simulink model "inverse_kinematics_simulation_with_y_pose"  (R2014a)
settings: Solver=ode45  StartTime=0.0  StopTime=inf  RelTol=1e-3
values from neighbouring files (symbols this model uses):
  h1 = y(:,1)    [initial_conditions.m]    (also in inverse_kinematics.m)
  h2 = z(:,2)    [initial_conditions.m]    (also in inverse_kinematics.m)
  h3 = x(:,3)    [initial_conditions.m]    (also in inverse_kinematics.m)
  h4 = z(:,4)    [initial_conditions.m]    (also in inverse_kinematics.m)
  h5 = x(:,5)    [initial_conditions.m]    (also in inverse_kinematics.m)
  h6 = x(:,6)    [initial_conditions.m]    (also in inverse_kinematics.m)
  h7 = y(:,7)    [initial_conditions.m]    (also in inverse_kinematics.m)
  sampling_time = 0.01    [initial_conditions.m]
libraries: vrlib x1
settings Model: Creator=İSMAİL  LastModifiedBy=İSMAİL

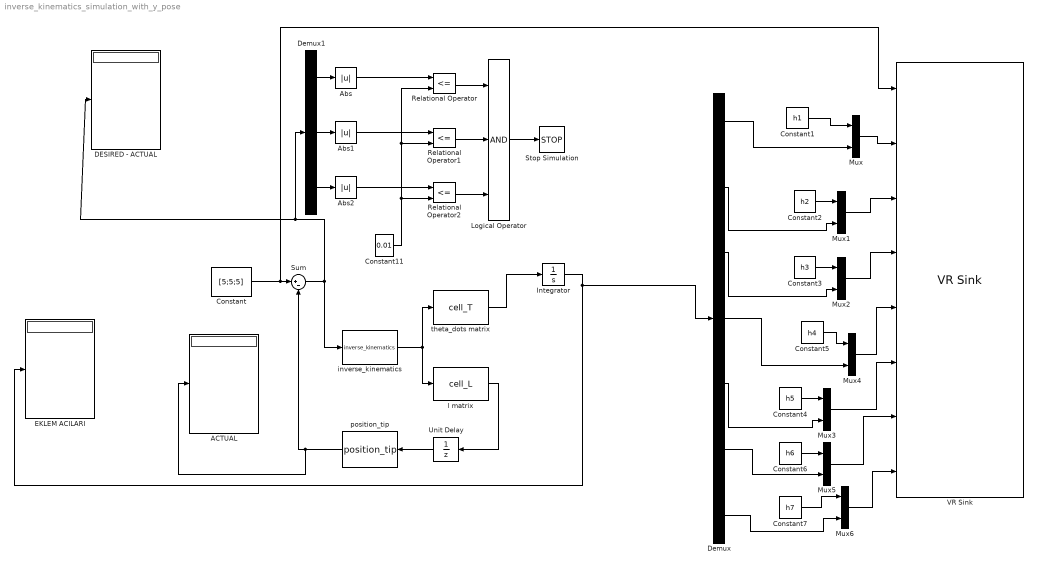
== system inverse_kinematics_simulation_with_y_pose ==
  ACTUAL : Display
  Abs : Abs
  Abs1 : Abs
  Abs2 : Abs
  Constant : Constant  Value=[5;5;5]  VectorParams1D=off
  Constant1 : Constant  Value=h1  VectorParams1D=off
  Constant11 : Constant  Value=0.01  VectorParams1D=off
  Constant2 : Constant  Value=h2  VectorParams1D=off
  Constant3 : Constant  Value=h3  VectorParams1D=off
  Constant4 : Constant  Value=h5  VectorParams1D=off
  Constant5 : Constant  Value=h4  VectorParams1D=off
  Constant6 : Constant  Value=h6  VectorParams1D=off
  Constant7 : Constant  Value=h7  VectorParams1D=off
  DESIRED - ACTUAL : Display
  Demux : Demux  Outputs=7
  Demux1 : Demux  Outputs=3
  EKLEM ACILARI : Display
  Integrator : Integrator
  Logical Operator : Logic  Inputs=3  AllPortsSameDT=off  OutDataTypeStr=boolean
  Mux{,1..6} (7 alike) : Mux  Inputs=2
  Relational Operator : RelationalOperator  Operator=<=  OutDataTypeStr=boolean
  Relational Operator1 : RelationalOperator  Operator=<=  OutDataTypeStr=boolean
  Relational Operator2 : RelationalOperator  Operator=<=  OutDataTypeStr=boolean
  Stop Simulation : Stop
  Sum : Sum  Inputs=|+-
  Unit Delay : UnitDelay  SampleTime=-1
  VR Sink : vrlib/VR Sink  InstantiateOnLoad=on  SampleTime=-1  ViewEnable=on  RemoteChange=off  RemoteView=off  FieldsWritten=Target.translation.3.1.1.double#Joint1.rotation.4.1.1.double#Joint2.rotation.4.1.1.double#Joint3.rotation.4.1.1.double#Joint4.rotation.4.1.1.double#Joint5.rotation.4.1.1.double#Joint6.rotation.4.1.1.double#Joint7.rotation.4.1.1.double  WorldFileName=vrml_y_pose.WRL  AutoView=off  VideoDimensions=[]  AllowVariableSize=off
  "inverse_kinematics " : MATLABFcn  MATLABFcn=inverse_kinematics  Output1D=off  SampleTime=sampling_time
  l matrix : MATLABFcn  MATLABFcn=cell_L  OutputDimensions=[24 7]  Output1D=off
  position_tip : MATLABFcn  MATLABFcn=position_tip  Output1D=off
  theta_dots matrix : MATLABFcn  MATLABFcn=cell_T  OutputDimensions=[7 1]  Output1D=off
  wires:
  position_tip/1 -> ACTUAL/1, Sum/2
  Integrator/1 -> EKLEM ACILARI/1, Demux/1
  Sum/1 -> Demux1/1, DESIRED - ACTUAL/1, "inverse_kinematics "/1
  "inverse_kinematics "/1 -> theta_dots matrix/1, l matrix/1
  theta_dots matrix/1 -> Integrator/1
  Constant2/1 -> Mux1/1
  Constant3/1 -> Mux2/1
  Constant4/1 -> Mux3/1
  Constant6/1 -> Mux5/1
  Constant7/1 -> Mux6/1
  Unit Delay/1 -> position_tip/1
  l matrix/1 -> Unit Delay/1
  Demux1/1 -> Abs/1
  Demux1/2 -> Abs1/1
  Demux1/3 -> Abs2/1
  Abs/1 -> Relational Operator/1
  Abs1/1 -> Relational Operator1/1
  Abs2/1 -> Relational Operator2/1
  Constant11/1 -> Relational Operator2/2, Relational Operator1/2, Relational Operator/2
  Relational Operator/1 -> Logical Operator/1
  Relational Operator1/1 -> Logical Operator/2
  Relational Operator2/1 -> Logical Operator/3
  Logical Operator/1 -> Stop Simulation/1
  Constant/1 -> Sum/1, VR Sink/1
  Constant1/1 -> Mux/1
  Constant5/1 -> Mux4/1
  Mux/1 -> VR Sink/2
  Mux1/1 -> VR Sink/3
  Mux2/1 -> VR Sink/4
  Mux4/1 -> VR Sink/5
  Mux3/1 -> VR Sink/6
  Mux5/1 -> VR Sink/7
  Mux6/1 -> VR Sink/8
  Demux/1 -> Mux/2
  Demux/2 -> Mux1/2
  Demux/3 -> Mux2/2
  Demux/4 -> Mux4/2
  Demux/5 -> Mux3/2
  Demux/6 -> Mux5/2
  Demux/7 -> Mux6/2
